simulink model "shipRdelta_sin"  (Simulink 8.3)
settings: Solver=ode3  StartTime=0.0  StopTime=1500  FixedStep=0.3  RelTol=1e-3
libraries: simulink x1
settings Model: Creator=Administrator  LastModifiedBy=jackyjing
settings OptimizationCC: ExpressionDepthLimit=2147483647
settings DebuggingCC: FcnCallInpInsideContextMsg=UseLocalSettings

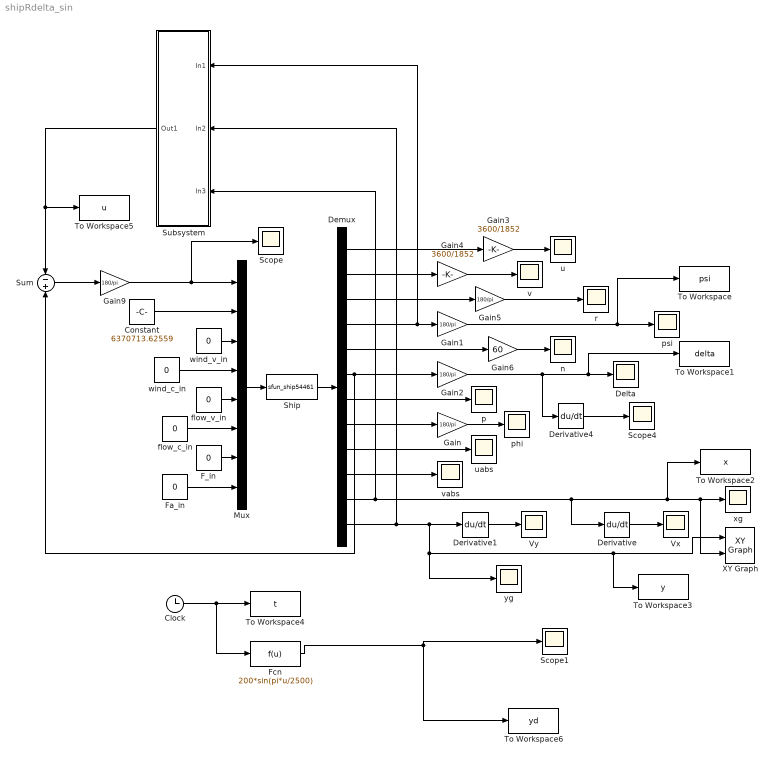
== system shipRdelta_sin ==
  Clock : Clock
  Constant : Constant  Value=6370713.62559
  Delta : Scope
      settings: TickLabels=on  TimeRange=1500  YMin=-35  YMax=35  SaveName=ScopeData5
  Demux : Demux  Outputs=12
  Derivative : Derivative
  Derivative1 : Derivative
  Derivative4 : Derivative
  F_in : Constant  Value=0
  Fa_in : Constant  Value=0
  Fcn : Fcn  Expr=200*sin(pi*u/2500)
  Gain{,1..2,5,9} (5 alike) : Gain  Gain=180/pi
  Gain3 : Gain  Gain=3600/1852
  Gain4 : Gain  Gain=3600/1852
  Gain6 : Gain  Gain=60
  Mux : Mux  Inputs=8
  Scope : Scope
      settings: TimeRange=1000  YMin=-0.6  YMax=0.8  SaveName=ScopeData14
  Scope1 : Scope
      settings: YMin=-700  YMax=700  SaveName=ScopeData18
  Scope4 : Scope
      settings: YMin=-0.005  YMax=0.002  SaveName=ScopeData15
  Ship : S-Function  FunctionName=sfun_ship54461  EnableBusSupport=off
  Subsystem : Subsystem
  Sum : Sum  Inputs=-|+
  To Workspace : ToWorkspace  VariableName=psi  SampleTime=-1
  To Workspace1 : ToWorkspace  VariableName=delta  SampleTime=-1
  To Workspace2 : ToWorkspace  VariableName=x  SampleTime=-1
  To Workspace3 : ToWorkspace  VariableName=y  SampleTime=-1
  To Workspace4 : ToWorkspace  VariableName=t  SampleTime=-1
  To Workspace5 : ToWorkspace  VariableName=u  SampleTime=-1
  To Workspace6 : ToWorkspace  VariableName=yd  SampleTime=-1
  "Vx " : Scope
      settings: TickLabels=on  SaveName=ScopeData8
  Vy : Scope
      settings: TickLabels=on  SaveName=ScopeData9
  XY Graph : simulink/Sinks/XY Graph  xmin=-1000  xmax=20000  ymin=-2000  ymax=2000  st=-1
  flow_c_in : Constant  Value=0
  flow_v_in : Constant  Value=0
  n : Scope
      settings: TickLabels=on  YMin=38.5  YMax=46.5  SaveName=ScopeData4
  p : Scope
      settings: TickLabels=on  SaveName=ScopeData10
  phi : Scope
      settings: YMin=-0.00175  YMax=0.0015  SaveName=ScopeData11
  psi : Scope
      settings: TickLabels=on  TimeRange=500  YMin=9.9825  YMax=10.01  SaveName=ScopeData3
  r : Scope
      settings: TickLabels=on  SaveName=ScopeData2
  u : Scope
      settings: TickLabels=on  YMin=15.075  YMax=15.625
  uabs : Scope
      settings: TickLabels=on  YMin=10.75  YMax=15  SaveName=ScopeData6
  v : Scope
      settings: TickLabels=on  YMin=-0.3  YMax=0.15
  vabs : Scope
      settings: TickLabels=on  YMin=-1.75  YMax=0  SaveName=ScopeData7
  wind_c_in : Constant  Value=0
  wind_v_in : Constant  Value=0
  xg : Scope
      settings: TickLabels=on  YMin=-300  YMax=900  SaveName=ScopeData12
  yg : Scope
      settings: TickLabels=on  YMin=250  YMax=475  SaveName=ScopeData13
  wires:
  Ship/1 -> Demux/1
  Demux/1 -> Gain3/1
  Demux/2 -> Gain4/1
  Demux/3 -> Gain5/1
  Demux/5 -> Gain6/1
  Demux/6 -> Sum/2, Gain2/1
  Demux/7 -> p/1
  Demux/8 -> Gain/1
  Gain1/1 -> psi/1, To Workspace/1
  Gain/1 -> phi/1
  Gain3/1 -> u/1
  Gain4/1 -> v/1
  Gain5/1 -> r/1
  Gain6/1 -> n/1
  Demux/9 -> uabs/1
  Demux/10 -> vabs/1
  Demux/12 -> Derivative1/1, yg/1, XY Graph/1, To Workspace3/1, Subsystem/2(In2)
  Demux/11 -> Subsystem/3(In3), Derivative/1, xg/1, XY Graph/2, To Workspace2/1
  Derivative/1 -> "Vx "/1
  Derivative1/1 -> Vy/1
  wind_v_in/1 -> Mux/3
  wind_c_in/1 -> Mux/4
  flow_v_in/1 -> Mux/5
  F_in/1 -> Mux/7
  Fa_in/1 -> Mux/8
  flow_c_in/1 -> Mux/6
  Mux/1 -> Ship/1
  Constant/1 -> Mux/2
  Sum/1 -> Gain9/1
  Derivative4/1 -> Scope4/1
  Subsystem/1(Out1) -> Sum/1, To Workspace5/1
  Demux/4 -> Gain1/1, Subsystem/1(In1)
  Gain2/1 -> Derivative4/1, Delta/1, To Workspace1/1
  Gain9/1 -> Mux/1, Scope/1
  Clock/1 -> Fcn/1, To Workspace4/1
  Fcn/1 -> To Workspace6/1, Scope1/1

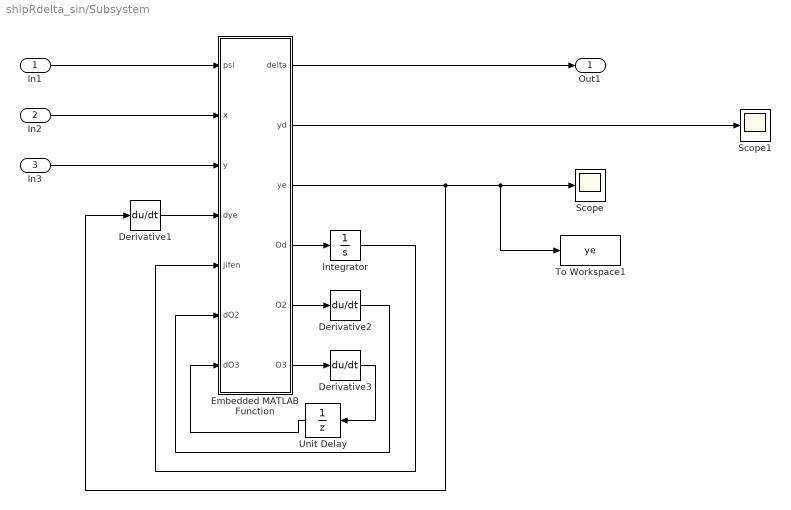
== system shipRdelta_sin/Subsystem ==
  In1 : Inport
  In2 : Inport  Port=2
  In3 : Inport  Port=3
  Derivative1 : Derivative
  Derivative2 : Derivative
  Derivative3 : Derivative
  Embedded MATLAB Function : MATLAB Function  TreatAsAtomicUnit=on
  Integrator : Integrator
  Scope : Scope
      settings: YMin=-50  YMax=950  SaveName=ScopeData16
  Scope1 : Scope
      settings: YMin=-700  YMax=700  SaveName=ScopeData17
  To Workspace1 : ToWorkspace  VariableName=ye  SampleTime=-1
  Unit Delay : UnitDelay  SampleTime=-1
  Out1 : Outport
  wires:
  Embedded MATLAB Function/6(O3) -> Derivative3/1
  Derivative3/1 -> Unit Delay/1
  Embedded MATLAB Function/5(O2) -> Derivative2/1
  Derivative2/1 -> Embedded MATLAB Function/6(dO2)
  Integrator/1 -> Embedded MATLAB Function/5(jifen)
  Embedded MATLAB Function/1(delta) -> Out1/1
  Embedded MATLAB Function/4(Od) -> Integrator/1
  In1/1 -> Embedded MATLAB Function/1(psi)
  In2/1 -> Embedded MATLAB Function/2(x)
  In3/1 -> Embedded MATLAB Function/3(y)
  Embedded MATLAB Function/3(ye) -> Derivative1/1, To Workspace1/1, Scope/1
  Derivative1/1 -> Embedded MATLAB Function/4(dye)
  Unit Delay/1 -> Embedded MATLAB Function/7(dO3)
  Embedded MATLAB Function/2(yd) -> Scope1/1

== matlab function Subsystem/Embedded MATLAB Function ==
  data: psi input double; x input double; y input double; dye input double; delta output double; yd output double; ye output double; Od output double; O2 output double; O3 output double; jifen input double; dO2 input double; dO3 input double
function [delta,yd,ye,Od,O2,O3] = fcn(psi,x,y,dye,jifen,dO2,dO3)
%K0=0.001;K1=15;K2=0.9;K3=0.01;K4=0.025;K5=0.25;Te=2.5;%可用
K0=0.001;K1=15;K2=1;K3=0.0005;K4=0.02;K5=20000;Te=2.5;
yd=500*sin(pi*x/2500);
ye=y-yd;


O1=K1*f(K0*ye)+dye;
Od=f(O1);
O2=psi+K2*jifen;
O3=K3*f(O2)+dO2;
O4=K4*f(O3)+dO3;
delta=-Te*K5*O4;

function mean=f(a)
mean=tanh(a);
% function mean=f(a)
% if(a<0.1&&a>-0.1)
%     mean=a;
% else 
%  mean=coth(a)-1/a;
% end
